simulink model "bumpy_road"  (R2020b)
settings: Solver=VariableStepAuto  StartTime=0.0  StopTime=100  RelTol=1e-3
values from neighbouring files (symbols this model uses):
  b = 40    [variable_declaration.m]
  k1 = 0.4    [variable_declaration.m]
  k2 = 0.6    [variable_declaration.m]
  m1 = 200    [variable_declaration.m]
  m2 = 20    [variable_declaration.m]
settings Model: Creator=shraddha  LastModifiedBy=shraddha

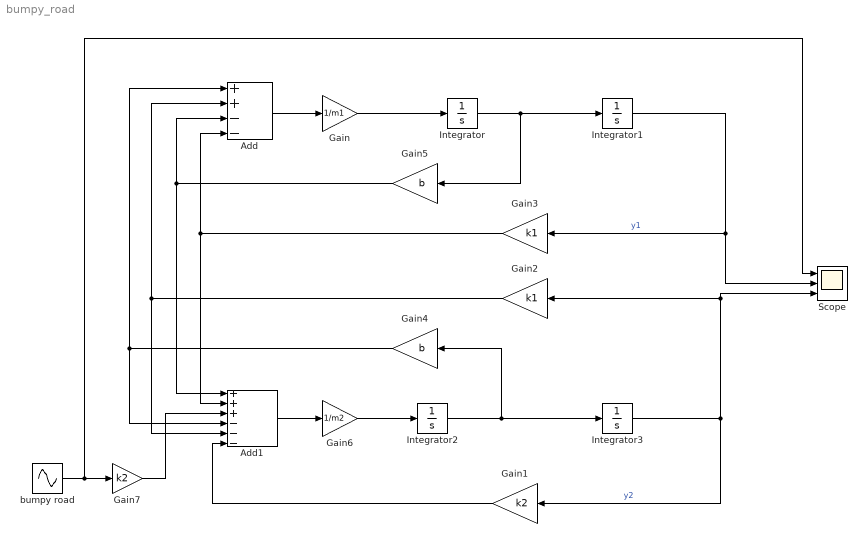
== system bumpy_road ==
  Add : Sum  Inputs=++--
  Add1 : Sum  Inputs=+++---
  Gain : Gain  Gain=1/m1
  Gain1 : Gain  Gain=k2
  Gain2 : Gain  Gain=k1
  Gain3 : Gain  Gain=k1
  Gain4 : Gain  Gain=b
  Gain5 : Gain  Gain=b
  Gain6 : Gain  Gain=1/m2
  Gain7 : Gain  Gain=k2
  Integrator{,1..3} (4 alike) : Integrator
  Scope : Scope  NumInputPorts=3
  bumpy road : Sin  Amplitude=0.2  Frequency=0.5  SampleTime=0
  wires:
  Add/1 -> Gain/1
  Gain/1 -> Integrator/1
  Integrator/1 -> Gain5/1, Integrator1/1
  Integrator1/1 -> Gain3/1, Scope/2  "y1"
  Integrator3/1 -> Gain1/1, Gain2/1, Scope/3  "y2"
  Integrator2/1 -> Gain4/1, Integrator3/1
  Gain6/1 -> Integrator2/1
  Add1/1 -> Gain6/1
  Gain4/1 -> Add1/4, Add/1
  Gain5/1 -> Add1/1, Add/3
  Gain2/1 -> Add1/5, Add/2
  Gain3/1 -> Add/4, Add1/2
  Gain1/1 -> Add1/6
  Gain7/1 -> Add1/3
  bumpy road/1 -> Scope/1, Gain7/1
